simulink model "ee_bldc_ideal_input_performance_curves"  (R2021a)
settings: Solver=ode14x  StartTime=0.0  StopTime=20  FixedStep=Ts  RelTol=1e-3
PreLoadFcn:
  | ee_bldc_ideal_input_performance_curves_data;
StopFcn:
  | ee_addSimlogTimeStamp(bdroot)
model workspace (MAT data in the model file):
  Ts = 5e-06
values from neighbouring files (symbols this model uses):
  Jm = results.Jm    [find_index_of_values.m]    (also in plot_BLDC_Design_space.m; simulate_design_space.m; testfile.m)
  Ke = results.Ke    [find_index_of_values.m]    (also in plot_BLDC_Design_space.m; simulate_design_space.m; testfile.m)
  No = results.N0_load_speed    [find_index_of_values.m]    (also in plot_BLDC_Design_space.m; simulate_design_space.m; testfile.m)
  nPolePairs = results.nPolePairs    [find_index_of_values.m]    (also in plot_BLDC_Design_space.m; simulate_design_space.m; testfile.m)
undefined symbols (not defined in the file or in its folder): DiscIntNeverNeededParam
libraries: fl_lib x35, nesl_utility x11, ee_lib x3, simulink x2, dspstat3 x2
CloseFcn:
  | try,close(h1_ee_bldc_ideal_input_performance_curves),end
  | clear h1_ee_bldc_ideal_input_performance_curves
  | 
  | clear pm_flux_linkage theta_constant nPolePairs
  | clear Ld Lq L0 Rs J lam Jsys Ts
  | 
  | clear currents efficiencys powers speeds torques
Description:
  | Calculate Performance Curves of BLDC
settings Model: SimulationMode=accelerator  OrderedModelArguments=off  Creator=The MathWorks, Inc.  LastModifiedBy=LenosBlueSky
settings SolverCC: AlgebraicLoopSolver=TrustRegion
settings DataIOCC: SaveTime=off  ReturnWorkspaceOutputs=off
settings DebuggingCC: SFMachineParentedDataDiag=warning  ArithmeticOperatorsInVariantConditions=warning

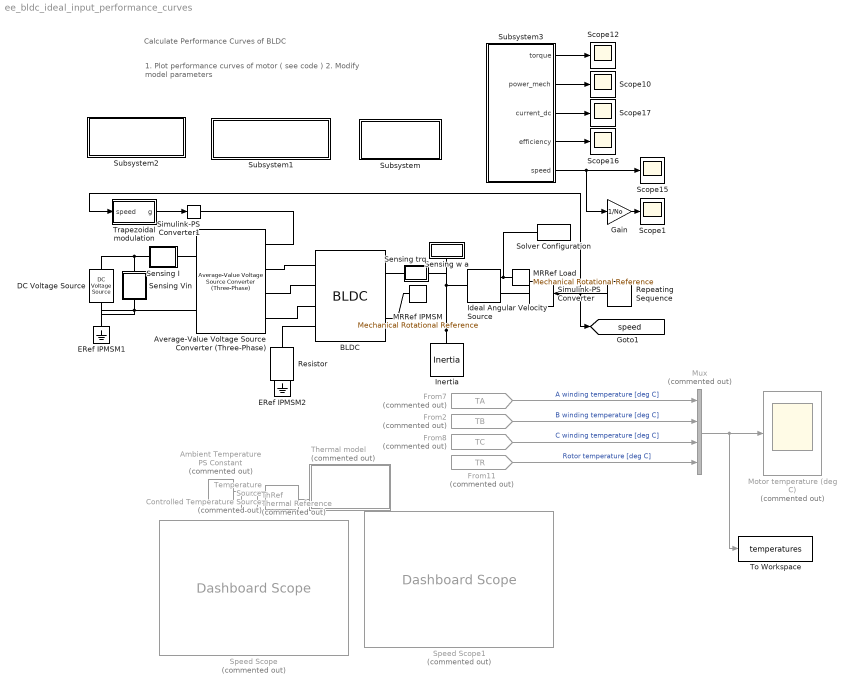
== system ee_bldc_ideal_input_performance_curves ==
  note: 1. Plot performance curves of motor ( see code )
      | 2. Modify model parameters
  note: Calculate Performance Curves of BLDC
  Ambient Temperature : fl_lib/Physical Signals/Sources/PS Constant  Commented=on  constant=300.15 K
  Average-Value Voltage Source Converter (Three-Phase) : ee_lib/Semiconductors & Converters/Converters/Average-Value Voltage Source Converter (Three-Phase)  losses_parameterization=ee.enum.converters.losses.fixed  Pfixed=1 W  ks=0.01  kc1=1.7 V  kc2=0.01 Ohm  Ploss_vect=[100, 800, 1870, 3250, 4900] W  Irms_vect=[10, 100, 200, 300, 400] A  Vdc_nom=300 V  thermal_mass=30000 J/K  temperature_specify=off  temperature_priority=High  temperature=298.15 K  temperature_nominal_specify=off  temperature_nominal_unit=K  temperature_nominal_value=1
      settings: SourceProductBaseCode=PS  InternalSimscapePortConfiguration="{\"Bottom\":[],\"Left\":[{\"id\":\"ModWave\",\"label\":\"ModWave\",\"type\":\"input\"},{\"id\":\"a\",\"label\":\"a\",\"type\":\"foundation.electrical.electrical\"},{\"id\":\"b\",\"label\":\"b\",\"type\":\"foundation.electrical.electrical\"},{\"id\":\"c\",\"label\":\"c\",\"type\":\"foundation.electrical.electrical\"}],\"Right\":[{\"id\":\"p\",\"label\":\"+\",\"type\":\"foundation.electrical.electrical\"},{\"id\":\"n\",\"label\":\"-\",\"type\":\"foundation.electrical.electrical\"}],\"Top\":[]}"
  BLDC : ee_lib/Electromechanical/Permanent Magnet/BLDC  winding_type=ee.enum.statorconnection.wye  rotor_param=2  pm_flux_linkage=Psi Wb  theta_constant=pi/(2*nPolePairs) rad  emf_max=No*2*pi*Ke/60 V  DphiDtheta_tab=0 Wb/rad  back_emf_tab=0 V  rotor_angle_tab=0 deg  w_meas=No rpm  nPolePairs=nPolePairs  stator_param=ee.enum.statorparam.LsLmMs  machine_param=ee.enum.dqparameterization.constant  Ld=Ld H  Lq=Lq H  idVec=[-200, 0, 200] A  iqVec=[-200, 0, 200] A  LdMatrix=0.00022 * ones(3, 3) H  LqMatrix=0.00022 * ones(3, 3) H  L0=L0 H  Ls=Ls H  Lm=0 H  Ms=Ms H  Rs=Rs Ohm  zero_sequence=ee.enum.park.zerosequence.include  J=Jm kg*m^2  lam=Bv N*m/(rad/s)  axes_param=1  i_d_specify=off  i_d_priority=None  i_d=0 A  i_d_nominal_specify=off  i_d_nominal_unit=A  i_d_nominal_value=1  i_q_specify=off  i_q_priority=None  i_q=0 A  i_q_nominal_specify=off  i_q_nominal_unit=A  i_q_nominal_value=1  torque_specify=off  torque_priority=None  torque=0 N*m  torque_nominal_specify=off  torque_nominal_unit=N*m  torque_nominal_value=1  angular_velocity_specify=off  angular_velocity_priority=High  angular_velocity=0 rpm  angular_velocity_nominal_specify=off  angular_velocity_nominal_unit=rpm  angular_velocity_nominal_value=1  angular_position_specify=off  angular_position_priority=High  angular_position=0 deg  angular_position_nominal_specify=off  angular_position_nominal_unit=deg  angular_position_nominal_value=1  loss_param=ee.enum.ironloss.none  losses_oc=[0, 0, 0] W  losses_sc=[0, 0, 0] W  f_losses=60 Hz  Isc_losses=95 A  Tmeas=298.15 K  alpha=3.93e-3 1/K  alpha_flux=-0.001 1/K  stator_thermal_mass=100 J/K  rotor_thermal_mass=200 J/K  Rm_percent_rotor=90  Rd_percent_rotor=30  temperatureA_specify=off  temperatureA_priority=High  temperatureA=25 degC  temperatureA_nominal_specify=off  temperatureA_nominal_unit=degC  temperatureA_nominal_value=1  temperatureB_specify=off  temperatureB_priority=High  temperatureB=25 degC  temperatureB_nominal_specify=off  temperatureB_nominal_unit=degC  temperatureB_nominal_value=1  temperatureC_specify=off  temperatureC_priority=High  temperatureC=25 degC  temperatureC_nominal_specify=off  temperatureC_nominal_unit=degC  temperatureC_nominal_value=1  temperatureR_specify=off  temperatureR_priority=High  temperatureR=25 degC  temperatureR_nominal_specify=off  temperatureR_nominal_unit=degC  temperatureR_nominal_value=1
      settings: SourceProductBaseCode=PS  InternalSimscapePortConfiguration="{\"Bottom\":[],\"Left\":[{\"id\":\"a\",\"label\":\"a\",\"type\":\"foundation.electrical.electrical\"},{\"id\":\"b\",\"label\":\"b\",\"type\":\"foundation.electrical.electrical\"},{\"id\":\"c\",\"label\":\"c\",\"type\":\"foundation.electrical.electrical\"},{\"id\":\"n\",\"label\":\"n\",\"type\":\"foundation.electrical.electrical\"}],\"Right\":[{\"id\":\"R\",\"label\":\"R\",\"type\":\"foundation.mechanical.rotational.rotational\"},{\"id\":\"C\",\"label\":\"C\",\"type\":\"foundation.mechanical.rotational.rotational\"}],\"Top\":[]}"
  DC Voltage Source : ee_lib/Additional Components/SPICE Sources/DC Voltage Source  DC=Vdc V
  ERef IPMSM1 : fl_lib/Electrical/Electrical Elements/Electrical Reference
  ERef IPMSM2 : fl_lib/Electrical/Electrical Elements/Electrical Reference
  From11 : From  Commented=on  GotoTag=TR  TagVisibility=global
  From2 : From  Commented=on  GotoTag=TB  TagVisibility=global
  From7 : From  Commented=on  GotoTag=TA  TagVisibility=global
  From8 : From  Commented=on  GotoTag=TC  TagVisibility=global
  Gain : Gain  Gain=1/No
  Ideal Angular Velocity Source : fl_lib/Mechanical/Mechanical Sources/Ideal Angular Velocity Source
  Inertia : fl_lib/Mechanical/Rotational Elements/Inertia  inertia=0.00201269 kg*m^2  num_ports=foundation.enum.numPorts2.one  w_specify=off  w_priority=High  w=0 rpm  w_nominal_specify=off  w_nominal_unit=rad/s  w_nominal_value=1  t_specify=off  t_priority=High  t=0 N*m  t_nominal_specify=off  t_nominal_unit=N*m  t_nominal_value=1
  MRRef IPMSM : fl_lib/Mechanical/Rotational Elements/Mechanical Rotational Reference
  MRRef Load : fl_lib/Mechanical/Rotational Elements/Mechanical Rotational Reference
  Motor temperature (deg C) : Scope  Commented=on
  Mux : Mux  Commented=on
  Repeating Sequence : simulink/Sources/Repeating Sequence  rep_seq_t=[0 2 20]  rep_seq_y=[0 1 1]*2*No
  Resistor : fl_lib/Electrical/Electrical Elements/Resistor  R=1e9 Ohm  i_specify=off  i_priority=None  i=0 A  i_nominal_specify=off  i_nominal_unit=A  i_nominal_value=1  v_specify=off  v_priority=None  v=0 V  v_nominal_specify=off  v_nominal_unit=V  v_nominal_value=1
  Scope{1,10,12,15..17} (6 alike) : Scope
  Sensing Vin : Subsystem
      mask Display:
      | disp('V')
      | port_label('Lconn',1,'+')
      | port_label('Rconn',1,'-')
  Sensing trq : Subsystem
      mask Display: disp('trq')
  Sensing w a : Subsystem
      mask Display: disp('w')
  Sensing I : Subsystem
      mask Display:
      | disp('idc')
      | port_label('Lconn',1,'+')
      | port_label('Rconn',1,'-')
  Simulink-PS Converter : nesl_utility/Simulink-PS Converter  PhysicalDomain=network_engine_domain  SubClassName=ps_input  LeftPortType=input  RightPortType=output  PseudoPeriodic=off  Frequencies=[]  NoiseDistribution=none  NoiseParameters=[]  Unit=rpm  AffineConversion=off  FilteringAndDerivatives=zero  SimscapeFilterOrder=1  InputFilterTimeConstant=0.001  UdotUserProvided=1
      settings: SourceProductBaseCode=PW,SS
  Simulink-PS Converter1 : nesl_utility/Simulink-PS Converter  PhysicalDomain=network_engine_domain  SubClassName=ps_input  LeftPortType=input  RightPortType=output  PseudoPeriodic=off  Frequencies=[]  NoiseDistribution=none  NoiseParameters=[]  Unit=1  AffineConversion=off  FilteringAndDerivatives=provide  SimscapeFilterOrder=1  InputFilterTimeConstant=0.001  UdotUserProvided=0
      settings: SourceProductBaseCode=PW,SS
  Solver Configuration : nesl_utility/Solver Configuration  PhysicalDomain=network_engine_domain  SubClassName=solver  LeftPortType=input  RightPortType=generic  Tones=[]  Harmonics=[]  SimulateNoise=off  Profile=off  UseLocalSampling=off  EnableSwitchedLinearOptims=on  FrequencyDomain=off  UseCCode=off  RelTol=0.001  AbsTol=1e-06  MinStep=1e-09  ToWorkspace=off  RevertToSquareIcSolve=off  NumHomotopyIterations=100  PhasorMode=off  PhasorModeNumHarmonics=1  DoDC=off  ResidualTolerance=1e-9  UseLocalSolver=on  LocalSolverChoice=NE_BACKWARD_EULER_ADVANCER  LocalSolverSampleTime=Ts  DoFixedCost=on  MaxNonlinIter=4  MaxModeIter=2  ComputeImpulses=off  ImpulseIterations=2  LinearAlgebra=auto  EquationFormulation=NE_TIME_EF  DelaysMemoryBudget=1024  AutomaticFiltering=off  FilteringTimeConstant=0.001  PartitionStorageMethod=AS_NEEDED  PartitionMemoryBudget=1024  PartitionMethod=FAST
      settings: SourceProductBaseCode=PW,SS
  Speed Scope : DashboardScope  Commented=on
  Speed Scope1 : DashboardScope  Commented=on
  Subsystem : Subsystem
      mask Display: disp('EFFICIENCY')
  Subsystem1 : Subsystem
      mask Display: disp('MECHANICAL POWER')
  Subsystem2 : Subsystem
      mask Display: disp('DC POWER')
  Subsystem3 : Subsystem
  Temperature Source : fl_lib/Thermal/Thermal Sources/Controlled Temperature Source  Commented=on
  ThRef : fl_lib/Thermal/Thermal Elements/Thermal Reference  Commented=on
  Thermal model : Subsystem  Tag=PublishSubsystem  Commented=on
  To Workspace : ToWorkspace  VariableName=temperatures  SaveFormat=Timeseries  SampleTime=-1
  Trapezoidal modulation : Subsystem
  tag scope: speed=global
  wires:
  Repeating Sequence/1 -> [speed], Trapezoidal modulation/1(speed), Simulink-PS Converter/1
  Subsystem3/1(torque) -> Scope12/1
  Subsystem3/2(power_mech) -> Scope10/1
  Subsystem3/3(current_dc) -> Scope17/1
  Subsystem3/4(efficiency) -> Scope16/1
  Subsystem3/5(speed) -> Gain/1, Scope15/1
  Trapezoidal modulation/1(g) -> Simulink-PS Converter1/1
  Gain/1 -> Scope1/1
  From7/1 -> Mux/1  "A winding temperature [deg C]"
  From2/1 -> Mux/2  "B winding temperature [deg C]"
  From8/1 -> Mux/3  "C winding temperature [deg C]"
  From11/1 -> Mux/4  "Rotor temperature [deg C]"
  Mux/1 -> To Workspace/1, Motor temperature (deg C)/1
  connections:
  Solver Configuration/RConn1 -- MRRef Load/LConn1 -- Ideal Angular Velocity Source/RConn2
  Inertia/LConn1 -- Sensing w a/LConn1 -- Sensing trq/RConn1 -- Ideal Angular Velocity Source/LConn1
  Ideal Angular Velocity Source/RConn1 -- Simulink-PS Converter/RConn1
  BLDC/RConn1 -- Sensing trq/LConn1
  BLDC/RConn2 -- MRRef IPMSM/LConn1
  Resistor/RConn1 -- ERef IPMSM2/LConn1
  BLDC/LConn4 -- Resistor/LConn1
  BLDC/LConn2 -- Average-Value Voltage Source Converter (Three-Phase)/LConn3
  BLDC/LConn3 -- Average-Value Voltage Source Converter (Three-Phase)/LConn4
  Simulink-PS Converter1/RConn1 -- Average-Value Voltage Source Converter (Three-Phase)/LConn1
  Sensing Vin/RConn1 -- ERef IPMSM1/LConn1 -- DC Voltage Source/RConn1 -- Average-Value Voltage Source Converter (Three-Phase)/RConn2
  Sensing I/LConn1 -- DC Voltage Source/LConn1 -- Sensing Vin/LConn1
  Sensing I/RConn1 -- Average-Value Voltage Source Converter (Three-Phase)/RConn1
  ThRef/LConn1 -- Temperature Source/RConn2
  Temperature Source/LConn1 -- Thermal model/LConn2
  Ambient Temperature/RConn1 -- Temperature Source/RConn1
  Average-Value Voltage Source Converter (Three-Phase)/LConn2 -- BLDC/LConn1

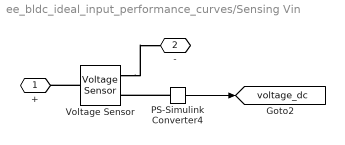
== system ee_bldc_ideal_input_performance_curves/Sensing Vin ==
  PS-Simulink Converter4 : nesl_utility/PS-Simulink Converter  PhysicalDomain=network_engine_domain  SubClassName=ps_output  LeftPortType=input  RightPortType=output  PseudoPeriodic=off  Frequencies=[]  Unit=V  AffineConversion=off
      settings: SourceProductBaseCode=PW,SS
  Voltage Sensor : fl_lib/Electrical/Electrical Sensors/Voltage Sensor
  + : PMIOPort  Side=Left
  - : PMIOPort  Port=2  Side=Right
  tag scope: voltage_dc=global
  wires:
  PS-Simulink Converter4/1 -> [voltage_dc]
  connections:
  Voltage Sensor/LConn1 -- +/RConn1
  Voltage Sensor/RConn2 -- -/RConn1
  PS-Simulink Converter4/LConn1 -- Voltage Sensor/RConn1

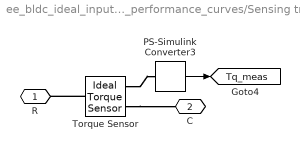
== system ee_bldc_ideal_input_performance_curves/Sensing trq ==
  PS-Simulink Converter3 : nesl_utility/PS-Simulink Converter  PhysicalDomain=network_engine_domain  SubClassName=ps_output  LeftPortType=input  RightPortType=output  PseudoPeriodic=off  Frequencies=[]  Unit=N*m  AffineConversion=off
      settings: SourceProductBaseCode=PW,SS
  Torque Sensor : fl_lib/Mechanical/Mechanical Sensors/Ideal Torque Sensor
  R : PMIOPort  Side=Left
  C : PMIOPort  Port=2  Side=Right
  tag scope: Tq_meas=global
  wires:
  PS-Simulink Converter3/1 -> [Tq_meas]
  connections:
  Torque Sensor/RConn1 -- C/RConn1
  Torque Sensor/RConn2 -- PS-Simulink Converter3/LConn1
  Torque Sensor/LConn1 -- R/RConn1

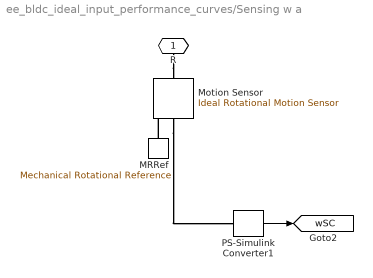
== system ee_bldc_ideal_input_performance_curves/Sensing w a ==
  MRRef : fl_lib/Mechanical/Rotational Elements/Mechanical Rotational Reference
  Motion Sensor : fl_lib/Mechanical/Mechanical Sensors/Ideal Rotational Motion Sensor  wrap_angle=simscape.enum.onoff.off  offset=0 deg
  PS-Simulink Converter1 : nesl_utility/PS-Simulink Converter  PhysicalDomain=network_engine_domain  SubClassName=ps_output  LeftPortType=input  RightPortType=output  PseudoPeriodic=off  Frequencies=[]  Unit=rad/s  AffineConversion=off
      settings: SourceProductBaseCode=PW,SS
  R : PMIOPort  Side=Left
  tag scope: wSC=global
  wires:
  PS-Simulink Converter1/1 -> [wSC]
  connections:
  R/RConn1 -- Motion Sensor/LConn1
  Motion Sensor/RConn2 -- PS-Simulink Converter1/LConn1
  MRRef/LConn1 -- Motion Sensor/RConn1

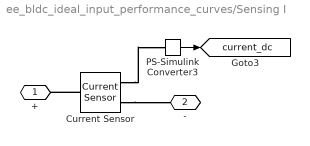
== system ee_bldc_ideal_input_performance_curves/Sensing I ==
  Current Sensor : fl_lib/Electrical/Electrical Sensors/Current Sensor
  PS-Simulink Converter3 : nesl_utility/PS-Simulink Converter  PhysicalDomain=network_engine_domain  SubClassName=ps_output  LeftPortType=input  RightPortType=output  PseudoPeriodic=off  Frequencies=[]  Unit=A  AffineConversion=off
      settings: SourceProductBaseCode=PW,SS
  + : PMIOPort  Side=Left
  - : PMIOPort  Port=2  Side=Right
  tag scope: current_dc=global
  wires:
  PS-Simulink Converter3/1 -> [current_dc]
  connections:
  Current Sensor/RConn2 -- -/RConn1
  Current Sensor/LConn1 -- +/RConn1
  Current Sensor/RConn1 -- PS-Simulink Converter3/LConn1

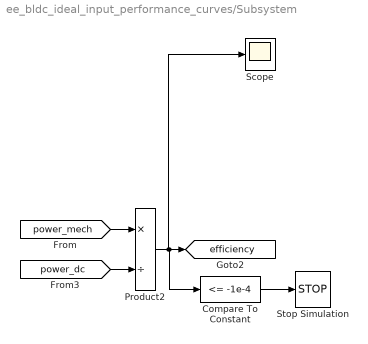
== system ee_bldc_ideal_input_performance_curves/Subsystem ==
  Compare To Constant : simulink/Logic and Bit Operations/Compare To Constant  relop=<=  const=-1e-4  OutDataTypeStr=boolean
  Product2 : Product  Inputs=*/
  Scope : Scope
  Stop Simulation : Stop
  tag scope: efficiency=global
  wires:
  [power_mech] -> Product2/1
  Product2/1 -> Scope/1, Compare To Constant/1, [efficiency]
  [power_dc] -> Product2/2
  Compare To Constant/1 -> Stop Simulation/1

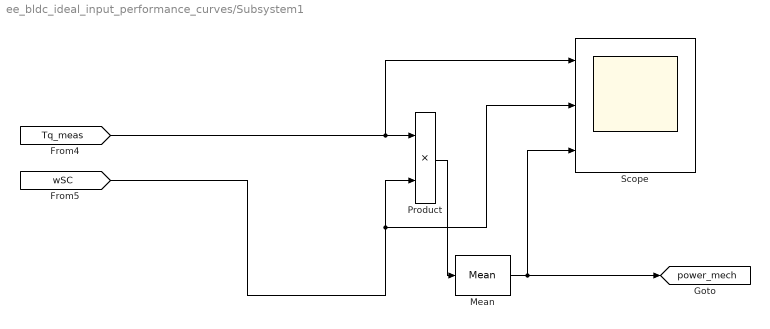
== system ee_bldc_ideal_input_performance_curves/Subsystem1 ==
  Mean : dspstat3/Mean  run=off  InputProcessing=Columns as channels (frame based)  reset_popup=None  directionMode=Each column  dimension=1  roiEnable=off  roiType=Rectangles  roiPortion=Entire ROI  roiOutput=Individual statistics for each ROI  roiFlag=off  roundingMode=Floor  overflowMode=off  outputDataTypeStr=Inherit: Same as accumulator  outputMin=[]  outputMax=[]  outputLastDataTypeStr=Inherit: Same as accumulator
  Product : Product
  Scope : Scope  NumInputPorts=3
  tag scope: power_mech=global
  wires:
  Product/1 -> Mean/1
  [Tq_meas] -> Product/1, Scope/1
  [wSC] -> Scope/2, Product/2
  Mean/1 -> [power_mech], Scope/3

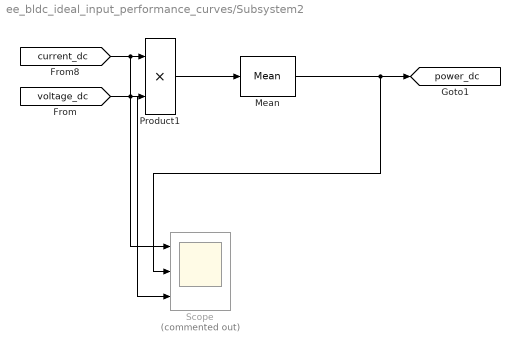
== system ee_bldc_ideal_input_performance_curves/Subsystem2 ==
  Mean : dspstat3/Mean  run=off  reset_popup=None  directionMode=Each column  dimension=1  roiEnable=off  roiType=Rectangles  roiPortion=Entire ROI  roiOutput=Individual statistics for each ROI  roiFlag=off  roundingMode=Floor  overflowMode=off  outputDataTypeStr=Inherit: Same as accumulator  outputMin=[]  outputMax=[]  outputLastDataTypeStr=Inherit: Same as accumulator
  Product1 : Product
  Scope : Scope  Commented=on  NumInputPorts=3
  tag scope: power_dc=global
  wires:
  Product1/1 -> Mean/1
  [voltage_dc] -> Scope/3, Product1/2
  [current_dc] -> Scope/1, Product1/1
  Mean/1 -> Scope/2, [power_dc]

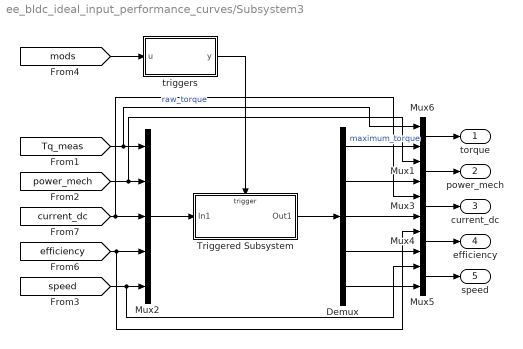
== system ee_bldc_ideal_input_performance_curves/Subsystem3 ==
  Demux : Demux  Outputs=5
  Mux{1,3..6} (5 alike) : Mux  Inputs=2
  Mux2 : Mux  Inputs=5
  Triggered Subsystem : Subsystem  TreatAsAtomicUnit=on
  triggers : Subsystem
  torque : Outport  VectorParamsAs1DForOutWhenUnconnected=off
  power_mech : Outport  Port=2  VectorParamsAs1DForOutWhenUnconnected=off
  current_dc : Outport  Port=3  VectorParamsAs1DForOutWhenUnconnected=off
  efficiency : Outport  Port=4  VectorParamsAs1DForOutWhenUnconnected=off
  speed : Outport  Port=5  VectorParamsAs1DForOutWhenUnconnected=off
  wires:
  triggers/1(y) -> Triggered Subsystem/Trigger
  [speed] -> Mux5/1, Mux2/5
  [mods] -> triggers/1(u)
  Triggered Subsystem/1(Out1) -> Demux/1
  [current_dc] -> Mux3/1, Mux2/3
  [efficiency] -> Mux4/1, Mux2/4
  [power_mech] -> Mux1/1, Mux2/2
  Mux2/1 -> Triggered Subsystem/1(In1)
  [Tq_meas] -> Mux6/1, Mux2/1  "raw_torque"
  Mux1/1 -> power_mech/1
  Mux3/1 -> current_dc/1
  Mux4/1 -> efficiency/1
  Demux/1 -> Mux6/2  "maximum_torque"
  Demux/2 -> Mux1/2
  Demux/3 -> Mux3/2
  Demux/4 -> Mux4/2
  Demux/5 -> Mux5/2
  Mux6/1 -> torque/1
  Mux5/1 -> speed/1

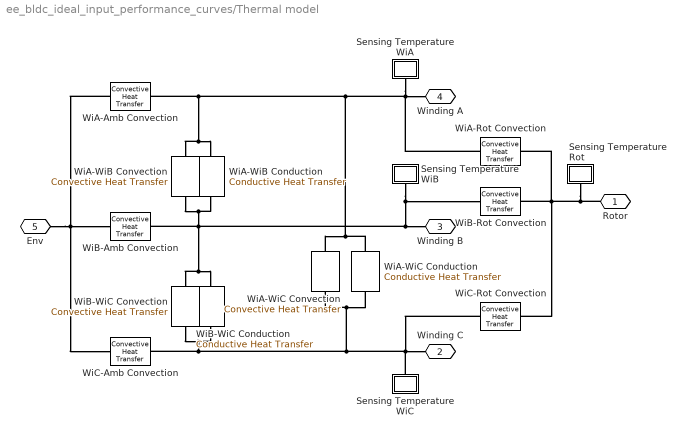
== system ee_bldc_ideal_input_performance_curves/Thermal model ==
  Sensing Temperature Rot : Subsystem
      mask Display: disp('TR')
  Sensing Temperature WiA : Subsystem
      mask Display: disp('TA')
  Sensing Temperature WiB : Subsystem
      mask Display: disp('TB')
  Sensing Temperature WiC : Subsystem
      mask Display: disp('TC')
  WiA-Amb Convection : fl_lib/Thermal/Thermal Elements/Convective Heat Transfer  area=0.1 m^2  heat_tr_coeff=20 W/(m^2 * K)  T_specify=off  T_priority=None  T=0 K  T_nominal_specify=off  T_nominal_unit=K  T_nominal_value=1  Q_specify=off  Q_priority=None  Q=0 J/s  Q_nominal_specify=off  Q_nominal_unit=J/s  Q_nominal_value=1
  WiA-Rot Convection : fl_lib/Thermal/Thermal Elements/Convective Heat Transfer  area=0.02 m^2  heat_tr_coeff=200 W/(m^2 * K)  T_specify=off  T_priority=None  T=0 K  T_nominal_specify=off  T_nominal_unit=K  T_nominal_value=1  Q_specify=off  Q_priority=None  Q=0 J/s  Q_nominal_specify=off  Q_nominal_unit=J/s  Q_nominal_value=1
  WiA-WiB Conduction : fl_lib/Thermal/Thermal Elements/Conductive Heat Transfer  area=0.002 m^2  thickness=0.1 m  th_cond=80 W/(m*K)  T_specify=off  T_priority=None  T=0 K  T_nominal_specify=off  T_nominal_unit=K  T_nominal_value=1  Q_specify=off  Q_priority=None  Q=0 J/s  Q_nominal_specify=off  Q_nominal_unit=J/s  Q_nominal_value=1
  WiA-WiB Convection : fl_lib/Thermal/Thermal Elements/Convective Heat Transfer  area=0.004 m^2  heat_tr_coeff=200 W/(m^2 * K)  T_specify=off  T_priority=None  T=0 K  T_nominal_specify=off  T_nominal_unit=K  T_nominal_value=1  Q_specify=off  Q_priority=None  Q=0 J/s  Q_nominal_specify=off  Q_nominal_unit=J/s  Q_nominal_value=1
  WiA-WiC Conduction : fl_lib/Thermal/Thermal Elements/Conductive Heat Transfer  area=0.002 m^2  thickness=0.1 m  th_cond=80 W/(m*K)  T_specify=off  T_priority=None  T=0 K  T_nominal_specify=off  T_nominal_unit=K  T_nominal_value=1  Q_specify=off  Q_priority=None  Q=0 J/s  Q_nominal_specify=off  Q_nominal_unit=J/s  Q_nominal_value=1
  WiA-WiC Convection : fl_lib/Thermal/Thermal Elements/Convective Heat Transfer  area=0.004 m^2  heat_tr_coeff=200 W/(m^2 * K)  T_specify=off  T_priority=None  T=0 K  T_nominal_specify=off  T_nominal_unit=K  T_nominal_value=1  Q_specify=off  Q_priority=None  Q=0 J/s  Q_nominal_specify=off  Q_nominal_unit=J/s  Q_nominal_value=1
  WiB-Amb Convection : fl_lib/Thermal/Thermal Elements/Convective Heat Transfer  area=0.1 m^2  heat_tr_coeff=20 W/(m^2 * K)  T_specify=off  T_priority=None  T=0 K  T_nominal_specify=off  T_nominal_unit=K  T_nominal_value=1  Q_specify=off  Q_priority=None  Q=0 J/s  Q_nominal_specify=off  Q_nominal_unit=J/s  Q_nominal_value=1
  WiB-Rot Convection : fl_lib/Thermal/Thermal Elements/Convective Heat Transfer  area=0.02 m^2  heat_tr_coeff=200 W/(m^2 * K)  T_specify=off  T_priority=None  T=0 K  T_nominal_specify=off  T_nominal_unit=K  T_nominal_value=1  Q_specify=off  Q_priority=None  Q=0 J/s  Q_nominal_specify=off  Q_nominal_unit=J/s  Q_nominal_value=1
  WiB-WiC Conduction : fl_lib/Thermal/Thermal Elements/Conductive Heat Transfer  area=0.002 m^2  thickness=0.1 m  th_cond=80 W/(m*K)  T_specify=off  T_priority=None  T=0 K  T_nominal_specify=off  T_nominal_unit=K  T_nominal_value=1  Q_specify=off  Q_priority=None  Q=0 J/s  Q_nominal_specify=off  Q_nominal_unit=J/s  Q_nominal_value=1
  WiB-WiC Convection : fl_lib/Thermal/Thermal Elements/Convective Heat Transfer  area=0.004 m^2  heat_tr_coeff=200 W/(m^2 * K)  T_specify=off  T_priority=None  T=0 K  T_nominal_specify=off  T_nominal_unit=K  T_nominal_value=1  Q_specify=off  Q_priority=None  Q=0 J/s  Q_nominal_specify=off  Q_nominal_unit=J/s  Q_nominal_value=1
  WiC-Amb Convection : fl_lib/Thermal/Thermal Elements/Convective Heat Transfer  area=0.1 m^2  heat_tr_coeff=20 W/(m^2 * K)  T_specify=off  T_priority=None  T=0 K  T_nominal_specify=off  T_nominal_unit=K  T_nominal_value=1  Q_specify=off  Q_priority=None  Q=0 J/s  Q_nominal_specify=off  Q_nominal_unit=J/s  Q_nominal_value=1
  WiC-Rot Convection : fl_lib/Thermal/Thermal Elements/Convective Heat Transfer  area=0.02 m^2  heat_tr_coeff=200 W/(m^2 * K)  T_specify=off  T_priority=None  T=0 K  T_nominal_specify=off  T_nominal_unit=K  T_nominal_value=1  Q_specify=off  Q_priority=None  Q=0 J/s  Q_nominal_specify=off  Q_nominal_unit=J/s  Q_nominal_value=1
  Rotor : PMIOPort  Side=Left
  Winding C : PMIOPort  Port=2  Side=Right
  Winding B : PMIOPort  Port=3  Side=Right
  Winding A : PMIOPort  Port=4  Side=Right
  Env : PMIOPort  Port=5  Side=Left
  connections:
  WiA-Rot Convection/RConn1 -- WiA-WiC Conduction/RConn1 -- WiA-WiC Convection/RConn1 -- WiA-WiB Convection/LConn1 -- WiA-WiB Conduction/LConn1 -- WiA-Amb Convection/LConn1 -- Sensing Temperature WiA/LConn1 -- Winding A/RConn1
  Rotor/RConn1 -- Sensing Temperature Rot/LConn1 -- WiC-Rot Convection/LConn1 -- WiB-Rot Convection/LConn1 -- WiA-Rot Convection/LConn1
  WiA-WiB Convection/RConn1 -- WiA-WiB Conduction/RConn1 -- Sensing Temperature WiB/LConn1 -- WiB-Rot Convection/RConn1 -- Winding B/RConn1 -- WiB-Amb Convection/LConn1 -- WiB-WiC Conduction/LConn1 -- WiB-WiC Convection/LConn1
  WiC-Rot Convection/RConn1 -- Winding C/RConn1 -- WiB-WiC Conduction/RConn1 -- WiB-WiC Convection/RConn1 -- WiC-Amb Convection/LConn1 -- WiA-WiC Convection/LConn1 -- WiA-WiC Conduction/LConn1 -- Sensing Temperature WiC/LConn1
  WiA-Amb Convection/RConn1 -- Env/RConn1 -- WiC-Amb Convection/RConn1 -- WiB-Amb Convection/RConn1

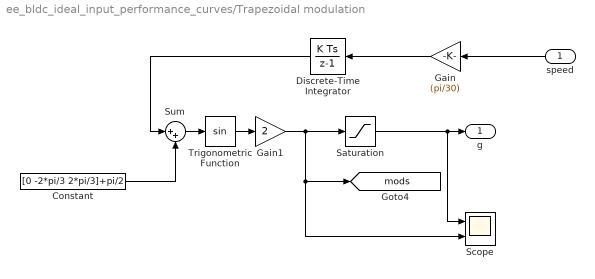
== system ee_bldc_ideal_input_performance_curves/Trapezoidal modulation ==
  speed : Inport
  Constant : Constant  Value=[0 -2*pi/3 2*pi/3]+pi/2
  Discrete-Time Integrator : DiscreteIntegrator  gainval=nPolePairs  SampleTime=-1  ICPrevOutput=DiscIntNeverNeededParam  ICPrevScaledInput=DiscIntNeverNeededParam
  Gain : Gain  Gain=(pi/30)
  Gain1 : Gain  Gain=2
  Saturation : Saturate  UpperLimit=1  LowerLimit=-1
  Scope : Scope  NumInputPorts=2
  Sum : Sum  Inputs=|++
  Trigonometric Function : Trigonometry
  g : Outport  VectorParamsAs1DForOutWhenUnconnected=off
  tag scope: mods=global
  wires:
  Trigonometric Function/1 -> Gain1/1
  Discrete-Time Integrator/1 -> Sum/1
  Gain1/1 -> Scope/2, [mods], Saturation/1
  Saturation/1 -> Scope/1, g/1
  Constant/1 -> Sum/2
  Sum/1 -> Trigonometric Function/1
  speed/1 -> Gain/1
  Gain/1 -> Discrete-Time Integrator/1

== system ee_bldc_ideal_input_performance_curves/Subsystem3/Triggered Subsystem ==
  In1 : Inport
  Trigger : TriggerPort  TriggerType=either  VariantControl=Variant
  Out1 : Outport  VectorParamsAs1DForOutWhenUnconnected=off
  wires:
  In1/1 -> Out1/1

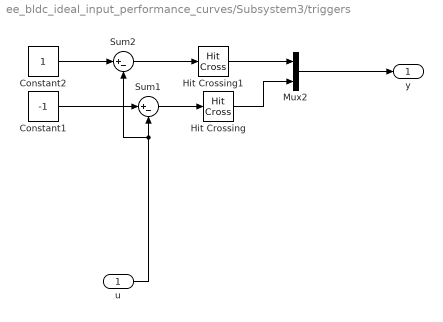
== system ee_bldc_ideal_input_performance_curves/Subsystem3/triggers ==
  u : Inport
  Constant1 : Constant  Value=-1
  Constant2 : Constant
  Hit Crossing : HitCross
  Hit Crossing1 : HitCross
  Mux2 : Mux  Inputs=2
  Sum1 : Sum  Inputs=|+-
  Sum2 : Sum  Inputs=|+-
  y : Outport  VectorParamsAs1DForOutWhenUnconnected=off
  wires:
  u/1 -> Sum2/2, Sum1/2
  Sum2/1 -> Hit Crossing1/1
  Hit Crossing/1 -> Mux2/2
  Sum1/1 -> Hit Crossing/1
  Constant1/1 -> Sum1/1
  Hit Crossing1/1 -> Mux2/1
  Constant2/1 -> Sum2/1
  Mux2/1 -> y/1

== system ee_bldc_ideal_input_performance_curves/Thermal model/Sensing Temperature Rot ==
  PS-Simulink Converter : nesl_utility/PS-Simulink Converter  PhysicalDomain=network_engine_domain  SubClassName=ps_output  LeftPortType=input  RightPortType=output  PseudoPeriodic=off  Frequencies=[]  Unit=degC  AffineConversion=on
      settings: SourceProductBaseCode=PW,SS
  Temperature Sensor : fl_lib/Thermal/Thermal Sensors/Temperature Sensor
  ThRef : fl_lib/Thermal/Thermal Elements/Thermal Reference
  H : PMIOPort  Side=Left
  tag scope: TR=global
  wires:
  PS-Simulink Converter/1 -> [TR]
  connections:
  Temperature Sensor/RConn2 -- PS-Simulink Converter/LConn1
  ThRef/LConn1 -- Temperature Sensor/RConn1
  H/RConn1 -- Temperature Sensor/LConn1

== system ee_bldc_ideal_input_performance_curves/Thermal model/Sensing Temperature WiA ==
  PS-Simulink Converter : nesl_utility/PS-Simulink Converter  PhysicalDomain=network_engine_domain  SubClassName=ps_output  LeftPortType=input  RightPortType=output  PseudoPeriodic=off  Frequencies=[]  Unit=degC  AffineConversion=on
      settings: SourceProductBaseCode=PW,SS
  Temperature Sensor : fl_lib/Thermal/Thermal Sensors/Temperature Sensor
  ThRef : fl_lib/Thermal/Thermal Elements/Thermal Reference
  H : PMIOPort  Side=Left
  tag scope: TA=global
  wires:
  PS-Simulink Converter/1 -> [TA]
  connections:
  H/RConn1 -- Temperature Sensor/LConn1
  ThRef/LConn1 -- Temperature Sensor/RConn1
  Temperature Sensor/RConn2 -- PS-Simulink Converter/LConn1

== system ee_bldc_ideal_input_performance_curves/Thermal model/Sensing Temperature WiB ==
  PS-Simulink Converter : nesl_utility/PS-Simulink Converter  PhysicalDomain=network_engine_domain  SubClassName=ps_output  LeftPortType=input  RightPortType=output  PseudoPeriodic=off  Frequencies=[]  Unit=degC  AffineConversion=on
      settings: SourceProductBaseCode=PW,SS
  Temperature Sensor : fl_lib/Thermal/Thermal Sensors/Temperature Sensor
  ThRef : fl_lib/Thermal/Thermal Elements/Thermal Reference
  H : PMIOPort  Side=Left
  tag scope: TB=global
  wires:
  PS-Simulink Converter/1 -> [TB]
  connections:
  Temperature Sensor/RConn2 -- PS-Simulink Converter/LConn1
  ThRef/LConn1 -- Temperature Sensor/RConn1
  H/RConn1 -- Temperature Sensor/LConn1

== system ee_bldc_ideal_input_performance_curves/Thermal model/Sensing Temperature WiC ==
  PS-Simulink Converter : nesl_utility/PS-Simulink Converter  PhysicalDomain=network_engine_domain  SubClassName=ps_output  LeftPortType=input  RightPortType=output  PseudoPeriodic=off  Frequencies=[]  Unit=degC  AffineConversion=on
      settings: SourceProductBaseCode=PW,SS
  Temperature Sensor : fl_lib/Thermal/Thermal Sensors/Temperature Sensor
  ThRef : fl_lib/Thermal/Thermal Elements/Thermal Reference
  H : PMIOPort  Side=Left
  tag scope: TC=global
  wires:
  PS-Simulink Converter/1 -> [TC]
  connections:
  H/RConn1 -- Temperature Sensor/LConn1
  ThRef/LConn1 -- Temperature Sensor/RConn1
  Temperature Sensor/RConn2 -- PS-Simulink Converter/LConn1
